simulink library "PCMULib"  (R2022b)
settings: Solver=ode45  StartTime=0.0  StopTime=10.0  RelTol=1e-3  EnableMultiTasking=on
undefined symbols (not defined in the file or in its folder): BreakpointData, BreakpointData1, BreakpointData2, BreakpointData_One_A, BreakpointData_Two_A, caaaa_dbi, caaaa_swi, cTmComprCtrl_n_i16SM4CmpHeatKiMax, cTmComprCtrl_n_i16SM4CmpHeatKiMin, cTmComprCtrl_n_i16SM4CmpHeatKpMax, cTmComprCtrl_n_i16SM4CmpHeatKpMin, cTmComprCtrl_Te_s32ErrCmpPIContinueHeatH, cTmComprCtrl_Te_s32ErrCmpPIContinueHeatL, cTmIn_n_ElacCmprReq_db, cTmIn_n_ElacCmprReq_sw, db, dbi, E2E_P01DataIDMode, E2E_P01ReceiverStatusType, EnumClass, iBit, initalValue, No_Runnable_Period, ObB_EidBsgStDerat_C, p_OVERRIDE_MASTER_SWITCH, SlDemoSign, sw, swi, SwitchOff_P, SwitchOn_P, Table, TableData_M, VCCTi33, VSysD_FidVehDerat1_C
libraries: simulink x22, CCMLib x11, simulink_need_slupdate x9, UXFD_Lib x7, canmsglib x2, PTCC_Lib x1, hdlsllib x1
(part 7 of 7)

== system PCMULib/Standard/Relation&Logic/RS_FF ==
  S : Inport
  R : Inport  Port=2
  AND : Logic  Operator=NOT  Inputs=1  AllPortsSameDT=off  OutDataTypeStr=boolean
  AND1 : Logic  AllPortsSameDT=off  OutDataTypeStr=boolean
  AND2 : Logic  Operator=OR  AllPortsSameDT=off  OutDataTypeStr=boolean
  Unit Delay : UnitDelay  SampleTime=-1  HasFrameUpgradeWarning=on
  Q : Outport
  wires:
  AND/1 -> AND1/1
  R/1 -> AND/1
  S/1 -> AND2/1
  AND2/1 -> AND1/2
  Unit Delay/1 -> AND2/2
  AND1/1 -> Q/1, Unit Delay/1

== system PCMULib/Standard/Relation&Logic/Relay ==
  In2 : Inport
  on : Inport  Port=2
  off : Inport  Port=3
  AND : Logic  Operator=NOT  Inputs=1  AllPortsSameDT=off  OutDataTypeStr=boolean
  AND1 : Logic  Operator=NOT  Inputs=1  AllPortsSameDT=off  OutDataTypeStr=boolean
  AND2 : Logic  AllPortsSameDT=off  OutDataTypeStr=boolean
  AND3 : Logic  Inputs=3  AllPortsSameDT=off  OutDataTypeStr=boolean
  AND4 : Logic  Operator=OR  AllPortsSameDT=off  OutDataTypeStr=boolean
  Relational Operator : RelationalOperator  Operator=<=  OutDataTypeStr=boolean  InputSameDT=off
  Relational Operator1 : RelationalOperator  Operator=<=  OutDataTypeStr=boolean  InputSameDT=off
  Unit Delay : UnitDelay  SampleTime=-1  HasFrameUpgradeWarning=on
  y : Outport
  wires:
  Relational Operator/1 -> AND1/1, AND2/1
  Relational Operator1/1 -> AND/1
  AND3/1 -> AND4/2
  AND4/1 -> Unit Delay/1, y/1
  AND/1 -> AND2/2, AND3/2
  on/1 -> Relational Operator/1
  In2/1 -> Relational Operator1/1, Relational Operator/2
  off/1 -> Relational Operator1/2
  AND2/1 -> AND4/1
  Unit Delay/1 -> AND3/3
  AND1/1 -> AND3/1

== system PCMULib/Standard/Relation&Logic/SignalDelay3 ==
  note: S T E A D Y
  note: D E L A Y
  note: H O L D
  note: T R I G
  note: C O U N T E R
  In1 : Inport
  tdOn : Inport  Port=2
  tdOff : Inport  Port=3
  AND : Logic  Operator=OR  AllPortsSameDT=off  OutDataTypeStr=boolean
  AND1 : Logic  AllPortsSameDT=off  OutDataTypeStr=boolean
  Add : Sum  SaturateOnIntegerOverflow=on
  Constant : Constant  Value=0  OutDataTypeStr=Inherit: Inherit via back propagation
  Constant1 : Constant  Value=0  OutDataTypeStr=Inherit: Inherit via back propagation
  Relational Operator : RelationalOperator  Operator===  OutDataTypeStr=boolean  InputSameDT=off
  Relational Operator1 : RelationalOperator  Operator=>  OutDataTypeStr=boolean  InputSameDT=off
  Relational Operator2 : RelationalOperator  OutDataTypeStr=boolean  InputSameDT=off
  Relational Operator3 : RelationalOperator  Operator===  OutDataTypeStr=boolean  InputSameDT=off
  Switch : Switch  Criteria=u2 ~= 0  Threshold=0.5  SaturateOnIntegerOverflow=off  InputSameDT=off
  Switch1 : Switch  Criteria=u2 ~= 0  Threshold=0.5  SaturateOnIntegerOverflow=off  InputSameDT=off
  Unit Delay : UnitDelay  SampleTime=-1  HasFrameUpgradeWarning=on
  Unit Delay1 : UnitDelay  SampleTime=-1  HasFrameUpgradeWarning=on
  Unit Delay2 : UnitDelay  SampleTime=-1  HasFrameUpgradeWarning=on
  ts : DataStoreRead  DataStoreName=ts  IndexOptions=Index vector (dialog)  Indices=1  OutputSizes=1
  y : Outport
  wires:
  Relational Operator2/1 -> AND/2
  Relational Operator1/1 -> AND1/2
  AND1/1 -> AND/1
  AND/1 -> Unit Delay2/1, Relational Operator3/2
  Unit Delay2/1 -> AND1/1
  Constant1/1 -> Relational Operator1/2
  ts/1 -> Add/2
  Relational Operator3/1 -> y/1
  Switch1/1 -> Relational Operator2/2
  tdOff/1 -> Switch1/3
  Constant/1 -> Switch/3
  Switch/1 -> Unit Delay/1, Relational Operator2/1, Relational Operator1/1
  Unit Delay1/1 -> Relational Operator/1
  In1/1 -> Relational Operator3/1, Unit Delay1/1, Switch1/2, Relational Operator/2
  Add/1 -> Switch/1
  Unit Delay/1 -> Add/1
  Relational Operator/1 -> Switch/2
  tdOn/1 -> Switch1/1

== system PCMULib/Standard/Relation&Logic/SignalTurnOffDelay ==
  note: True = 上面，cnt 清零
      | False = 下面 ，cnt 计数
  note: cnt 计数 < td,保持输出True
  u : Inport
  td : Inport  Port=2
  Add : Sum  SaturateOnIntegerOverflow=on
  Constant : Constant  Value=0
  Delay : Delay  DelayLength=1  InitialConditionSource=Input port  InitialCondition=0
      settings: InputPortMap=u0,p4
  Relational Operator : RelationalOperator  Operator=<=  OutDataTypeStr=boolean  InputSameDT=off
  Switch1 : Switch  Criteria=u2 ~= 0  Threshold=0.5  SaturateOnIntegerOverflow=off  InputSameDT=off
  ts : DataStoreRead  DataStoreName=ts  IndexOptions=Index vector (dialog)  Indices=1  OutputSizes=1
  y : Outport
  wires:
  Constant/1 -> Switch1/1
  Add/1 -> Switch1/3
  Relational Operator/1 -> y/1  "output"
  u/1 -> Switch1/2
  ts/1 -> Add/2
  Delay/1 -> Add/1
  Switch1/1 -> Delay/1, Relational Operator/1  "turnOffCnt"
  td/1 -> Delay/2, Relational Operator/2  "delay_td"

== system PCMULib/Standard/Relation&Logic/SignalTurnOnDelay ==
  u : Inport
  td : Inport  Port=2
  Add : Sum  SaturateOnIntegerOverflow=on
  Constant : Constant  Value=0  OutDataTypeStr=Inherit: Inherit via back propagation
  Relational Operator : RelationalOperator  Operator=>  OutDataTypeStr=boolean  InputSameDT=off
  Switch1 : Switch  Criteria=u2 ~= 0  Threshold=0.5  SaturateOnIntegerOverflow=off  InputSameDT=off
  Unit Delay : UnitDelay  SampleTime=-1  HasFrameUpgradeWarning=on
  ts : DataStoreRead  DataStoreName=ts  IndexOptions=Index vector (dialog)  Indices=1  OutputSizes=1
  y : Outport
  wires:
  ts/1 -> Add/2
  Unit Delay/1 -> Add/1
  td/1 -> Relational Operator/2
  Switch1/1 -> Unit Delay/1, Relational Operator/1
  Add/1 -> Switch1/1
  Constant/1 -> Switch1/3
  u/1 -> Switch1/2
  Relational Operator/1 -> y/1

== system PCMULib/Standard/Relation&Logic/SignalTurnOnOffDelay ==
  note: 1
  note: 0.01
  u : Inport
  td : Inport  Port=2
  Add : Sum  SaturateOnIntegerOverflow=on
  Delay : Delay  DelayLength=1  InitialConditionSource=Input port
      settings: InputPortMap=u0,p4
  Delay1 : Delay  DelayLength=1  InitialConditionSource=Input port
      settings: InputPortMap=u0,p4
  Relational Operator : RelationalOperator  Operator===  OutDataTypeStr=boolean  InputSameDT=off
  Relational Operator1 : RelationalOperator  Operator=>  OutDataTypeStr=boolean  InputSameDT=off
  Switch : Switch  Criteria=u2 ~= 0  Threshold=0.5  OutDataTypeStr=Inherit: Inherit via back propagation  SaturateOnIntegerOverflow=off  InputSameDT=off
  Switch1 : Switch  Criteria=u2 ~= 0  Threshold=0.5  SaturateOnIntegerOverflow=off  InputSameDT=off
  Unit Delay1 : UnitDelay  SampleTime=-1  HasFrameUpgradeWarning=on
  ts : DataStoreRead  DataStoreName=ts  IndexOptions=Index vector (dialog)  Indices=1  OutputSizes=1
  y : Outport
  wires:
  Switch1/1 -> Delay1/1, y/1
  Delay1/1 -> Switch1/3
  Relational Operator1/1 -> Switch1/2
  Relational Operator/1 -> Switch/2
  Add/1 -> Switch/1
  Switch/1 -> Unit Delay1/1, Relational Operator1/1
  td/1 -> Relational Operator1/2
  Unit Delay1/1 -> Add/1
  ts/1 -> Switch/3, Add/2
  u/1 -> Delay/1, Delay/2, Delay1/2, Switch1/1, Relational Operator/1
  Delay/1 -> Relational Operator/2

== system PCMULib/Standard/Relation&Logic/xbackground1 ==

== system PCMULib/Standard/Relation&Logic/xbackground2 ==

== system PCMULib/Standard/Relation&Logic/xbackground3 ==

== system PCMULib/Standard/Relation&Logic/xbackground4 ==

== system PCMULib/Standard/Relation&Logic/xbackground5 ==

== system PCMULib/Standard/Relation&Logic/xbackground6 ==

== system PCMULib/Standard/Relation&Logic/xbackground7 ==

== system PCMULib/Standard/Relation&Logic/xbackground8 ==

== system PCMULib/Standard/Relation&Logic/xbackground9 ==

== system PCMULib/Standard/Signals and systems/ESubsystem ==
  Enable_Name : EnablePort

== system PCMULib/Standard/Signals and systems/ETSubsystem ==
  Enable_Name : EnablePort
  Trigger_Name : TriggerPort  VariantControl=Variant

== system PCMULib/Standard/Signals and systems/Function-Call Subsystem ==
  In1 : Inport
  function : TriggerPort  TriggerType=function-call  VariantControl=Variant
  Out1 : Outport
  wires:
  In1/1 -> Out1/1

== system PCMULib/Standard/Signals and systems/Model Header ==

== system PCMULib/Standard/Signals and systems/RenameSignal ==
  Inport : Inport
  y : Outport
  wires:
  Inport/1 -> y/1

== system PCMULib/Standard/Signals and systems/Subsystem ==
  In1 : Inport
  Out1 : Outport
  wires:
  In1/1 -> Out1/1

== system PCMULib/Standard/Signals and systems/TSubsystem ==
  Trigger_Name : TriggerPort  VariantControl=Variant

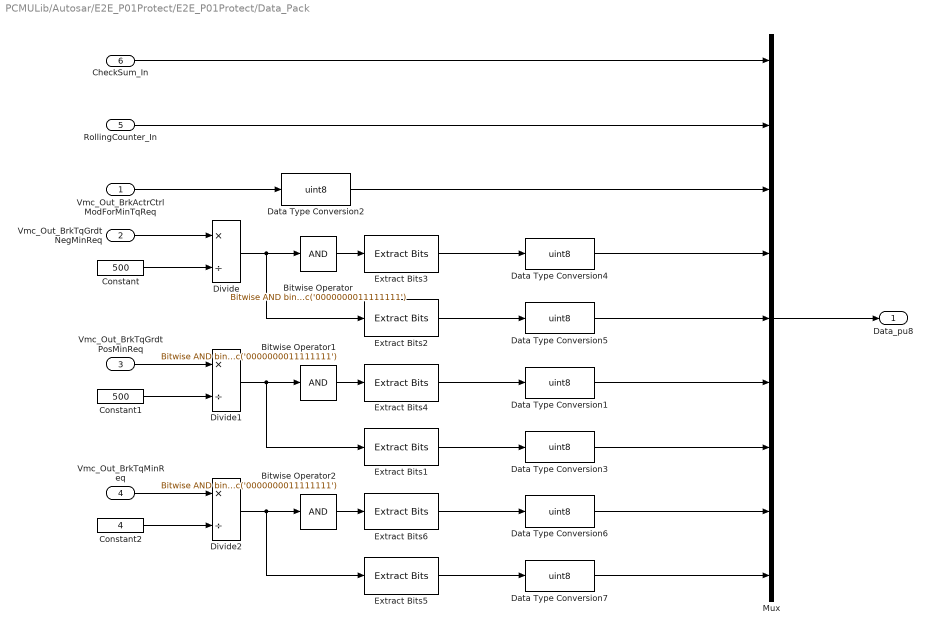
== system PCMULib/Autosar/E2E_P01Protect/E2E_P01Protect/Data_Pack ==
  Vmc_Out_BrkActrCtrlModForMinTqReq : Inport
  Vmc_Out_BrkTqGrdtNegMinReq : Inport  Port=2
  Vmc_Out_BrkTqGrdtPosMinReq : Inport  Port=3
  Vmc_Out_BrkTqMinReq : Inport  Port=4
  RollingCounter_In : Inport  Port=5
  CheckSum_In : Inport  Port=6
  Bitwise Operator : simulink/Logic and Bit Operations/Bitwise Operator  logicop=AND  UseBitMask=on  BitMask=bin2dec('0000000011111111')  BitMaskRealWorld=Stored Integer
  Bitwise Operator1 : simulink/Logic and Bit Operations/Bitwise Operator  logicop=AND  UseBitMask=on  BitMask=bin2dec('0000000011111111')  BitMaskRealWorld=Stored Integer
  Bitwise Operator2 : simulink/Logic and Bit Operations/Bitwise Operator  logicop=AND  UseBitMask=on  BitMask=bin2dec('0000000011111111')  BitMaskRealWorld=Stored Integer
  Constant : Constant  Value=500  OutDataTypeStr=uint16
      settings: CopyFcn=set_param(gcbh,'ShowName','off');
  Constant1 : Constant  Value=500  OutDataTypeStr=uint16
      settings: CopyFcn=set_param(gcbh,'ShowName','off');
  Constant2 : Constant  Value=4  OutDataTypeStr=uint8
      settings: CopyFcn=set_param(gcbh,'ShowName','off');
  Data Type Conversion{1..7} (7 alike) : DataTypeConversion  OutDataTypeStr=uint8  SaturateOnIntegerOverflow=off  RndMeth=Floor
  Divide : Product  Inputs=*/  OutDataTypeStr=uint16
  Divide1 : Product  Inputs=*/  OutDataTypeStr=uint16
  Divide2 : Product  Inputs=*/  OutDataTypeStr=uint16
  Extract Bits1 : simulink/Logic and Bit Operations/Extract Bits  bitsToExtract=Upper half  numBits=8  bitIdxRange=[0 7]  outScalingMode=Treat bit field as an integer
  Extract Bits2 : simulink/Logic and Bit Operations/Extract Bits  bitsToExtract=Upper half  numBits=8  bitIdxRange=[0 7]  outScalingMode=Treat bit field as an integer
  Extract Bits3 : simulink/Logic and Bit Operations/Extract Bits  bitsToExtract=Lower half  numBits=8  bitIdxRange=[0 7]  outScalingMode=Treat bit field as an integer
  Extract Bits4 : simulink/Logic and Bit Operations/Extract Bits  bitsToExtract=Lower half  numBits=8  bitIdxRange=[0 7]  outScalingMode=Treat bit field as an integer
  Extract Bits5 : simulink/Logic and Bit Operations/Extract Bits  bitsToExtract=Upper half  numBits=8  bitIdxRange=[0 7]  outScalingMode=Treat bit field as an integer
  Extract Bits6 : simulink/Logic and Bit Operations/Extract Bits  bitsToExtract=Lower half  numBits=8  bitIdxRange=[0 7]  outScalingMode=Treat bit field as an integer
  Mux : Mux  Inputs=9
  Data_pu8 : Outport
  wires:
  Mux/1 -> Data_pu8/1
  Vmc_Out_BrkActrCtrlModForMinTqReq/1 -> Data Type Conversion2/1
  Extract Bits3/1 -> Data Type Conversion4/1
  Constant/1 -> Divide/2
  Bitwise Operator/1 -> Extract Bits3/1
  Extract Bits2/1 -> Data Type Conversion5/1
  Divide/1 -> Extract Bits2/1, Bitwise Operator/1
  Vmc_Out_BrkTqGrdtNegMinReq/1 -> Divide/1
  Extract Bits4/1 -> Data Type Conversion1/1
  Constant1/1 -> Divide1/2
  Bitwise Operator1/1 -> Extract Bits4/1
  Extract Bits1/1 -> Data Type Conversion3/1
  Divide1/1 -> Extract Bits1/1, Bitwise Operator1/1
  Vmc_Out_BrkTqGrdtPosMinReq/1 -> Divide1/1
  Extract Bits6/1 -> Data Type Conversion6/1
  Constant2/1 -> Divide2/2
  Bitwise Operator2/1 -> Extract Bits6/1
  Extract Bits5/1 -> Data Type Conversion7/1
  Divide2/1 -> Extract Bits5/1, Bitwise Operator2/1
  Vmc_Out_BrkTqMinReq/1 -> Divide2/1
  RollingCounter_In/1 -> Mux/2
  CheckSum_In/1 -> Mux/1
  Data Type Conversion2/1 -> Mux/3
  Data Type Conversion4/1 -> Mux/4
  Data Type Conversion5/1 -> Mux/5
  Data Type Conversion1/1 -> Mux/6
  Data Type Conversion3/1 -> Mux/7
  Data Type Conversion6/1 -> Mux/8
  Data Type Conversion7/1 -> Mux/9

== system PCMULib/Autosar/E2E_P01Protect/E2E_P01Protect/E2E_Config ==
  DataLength : Inport
  DataID : Inport  Port=2
  BusCreator : BusCreator  Inputs=6  OutDataTypeStr=Bus: E2E_P01ConfigType  NonVirtualBus=on
      settings: CopyFcn=set_param(gcbh,'ShowName','off');  InheritFromInputs=off
  CRCOffset : Constant  Value=0  OutDataTypeStr=uint16
  CounterOffset : Constant  Value=8  OutDataTypeStr=uint16
  DataIDMode : simulink/Sources/Enumerated Constant  OutDataTypeStr=Enum: E2E_P01DataIDMode  Value=E2E_P01DataIDMode.E2E_P01_DATAID_BOTH  SampleTime=inf
  MaxDeltaCounterInit : Constant  Value=14  OutDataTypeStr=uint8
  E2E_P01_Config : Outport
  wires:
  DataID/1 -> BusCreator/2
  CounterOffset/1 -> BusCreator/6
  MaxDeltaCounterInit/1 -> BusCreator/4
  BusCreator/1 -> E2E_P01_Config/1
  DataIDMode/1 -> BusCreator/3
  DataLength/1 -> BusCreator/1
  CRCOffset/1 -> BusCreator/5

== system PCMULib/Autosar/E2E_P01Protect/E2E_P01Protect/E2E_P01Protect_S ==
  ConfigType : Inport
  SenderStateType : Inport  Port=2
  Data_pu8 : Inport  Port=3
  S-Function : S-Function  FunctionName=E2E_P01Protect_S  SFunctionDeploymentMode=off  EnableBusSupport=off
  Std_ReturnType : Outport
  wires:
  S-Function/1 -> Std_ReturnType/1
  Data_pu8/1 -> S-Function/3
  ConfigType/1 -> S-Function/1
  SenderStateType/1 -> S-Function/2

== system PCMULib/Autosar/E2E_P01_Check/E2E_Check/E2E_Check ==
  Status : Inport
  DataLength : Inport  Port=2
  DataID : Inport  Port=3
  AccrPedlNotCmpl_IsUpdated : Inport  Port=4
  CheckSum : Inport  Port=5
  RollingCounter : Inport  Port=6
  AccrPedlNotCmpl_Psd : Inport  Port=7
  AccrPedlNotCmpl_PsdSts : Inport  Port=8
  Data_ID_218 : Subsystem
  E2E_Config_ID_218 : Subsystem
  E2E_P01Check_S : Subsystem
      mask Display:
      | disp('E2E_P01Check');
      | port_label('input',1,'ConfigType');
      | port_label('input',2,'ReceiverStateType');
      | port_label('input',3,'Data_pu8');
      | port_label('output',1,'Std_ReturnType');
  E2E_P01ReceiverID_218 : Subsystem
  E2E_P01Check_ReturnType : Outport
  E2E_P01ReceiverStatus : Outport  Port=2
  wires:
  RollingCounter/1 -> Data_ID_218/2(RollingCounter)
  CheckSum/1 -> Data_ID_218/1(CheckSum)
  Data_ID_218/1(Data_pu8) -> E2E_P01Check_S/3(Data_pu8)
  E2E_P01Check_S/1(Std_ReturnType) -> E2E_P01Check_ReturnType/1
  E2E_Config_ID_218/1(E2E_Config_ID_218) -> E2E_P01Check_S/1(ConfigType)
  AccrPedlNotCmpl_IsUpdated/1 -> E2E_P01ReceiverID_218/1(AccrPedlNotCmpl_IsUpdated)
  DataLength/1 -> E2E_Config_ID_218/1(DataLength)
  E2E_P01ReceiverID_218/1(E2E_P01ReceiverState) -> E2E_P01ReceiverStatus/1, E2E_P01Check_S/2(ReceiverStateType)
  DataID/1 -> E2E_Config_ID_218/2(DataID)
  Status/1 -> E2E_P01ReceiverID_218/2(Status)
  AccrPedlNotCmpl_Psd/1 -> Data_ID_218/3(AccrPedlNotCmpl_Psd)
  AccrPedlNotCmpl_PsdSts/1 -> Data_ID_218/4(AccrPedlNotCmpl_PsdSts)

== system PCMULib/Calculation/PI/SaturationAndDeadband/absolute ==
  Input : Inport
  Compare To Constant2 : simulink/Logic and Bit Operations/Compare To Constant  relop=>=  const=0  OutDataTypeStr=boolean
  Constant10 : Constant  Value=0  OutDataTypeStr=Inherit: Inherit via back propagation
  Subtract : Sum  Inputs=-+  OutDataTypeStr=Inherit: Inherit via back propagation
  Switch10 : Switch  Criteria=u2 > Threshold  SaturateOnIntegerOverflow=off  InputSameDT=off
  Output : Outport  VectorParamsAs1DForOutWhenUnconnected=off
  wires:
  Constant10/1 -> Subtract/2
  Input/1 -> Subtract/1, Compare To Constant2/1, Switch10/1
  Subtract/1 -> Switch10/3
  Switch10/1 -> Output/1
  Compare To Constant2/1 -> Switch10/2

== system PCMULib/Custom/CAN/CanHex2Signed/condtion ==
  note: 判断条件:2^(n-1)-1
  note: 模：2^n
  bitL : Inport
  Add : Sum  Inputs=+-
      settings: CopyFcn=set_param(gcbh,'ShowName','off');
  Add1 : Sum  Inputs=+-
      settings: CopyFcn=set_param(gcbh,'ShowName','off');
  Constant : Constant  Value=2  OutDataTypeStr=single
      settings: CopyFcn=set_param(gcbh,'ShowName','off');
  Constant1 : Constant  OutDataTypeStr=single
      settings: CopyFcn=set_param(gcbh,'ShowName','off');
  Constant3 : Constant  OutDataTypeStr=uint8
      settings: CopyFcn=set_param(gcbh,'ShowName','off');
  Constant4 : Constant  Value=2  OutDataTypeStr=single
      settings: CopyFcn=set_param(gcbh,'ShowName','off');
  Gain : Gain  OutDataTypeStr=uint32
      settings: CopyFcn=set_param(gcbh,'ShowName','off');
  Math Function : Math  Operator=pow  SignedPower=on  OutputSignalType=real
  Math Function1 : Math  Operator=pow  SignedPower=on  OutputSignalType=real
  cond : Outport
  2^n : Outport  Port=2
  wires:
  Add/1 -> cond/1
  Gain/1 -> Add/1
  Constant4/1 -> Math Function1/1
  Add1/1 -> Math Function1/2
  Constant1/1 -> Add1/2
  Constant/1 -> Math Function/1
  Math Function/1 -> 2^n/1
  Math Function1/1 -> Gain/1
  Constant3/1 -> Add/2
  bitL/1 -> Math Function/2, Add1/1

== system PCMULib/Custom/CAN/CanHex2Signed/signal_conditioning ==
  note: 判断输入的BitLength是否（0<u1<=32bit）;
      | 并向下取整。
  In1 : Inport
  Constant1 : Constant  Value=0  OutDataTypeStr=single
      settings: CopyFcn=set_param(gcbh,'ShowName','off');
  Constant2 : Constant  Value=32  OutDataTypeStr=single
      settings: CopyFcn=set_param(gcbh,'ShowName','off');
  Constant4 : Constant  Value=32  OutDataTypeStr=single
      settings: CopyFcn=set_param(gcbh,'ShowName','off');
  Constant7 : Constant  Value=0  OutDataTypeStr=single
      settings: CopyFcn=set_param(gcbh,'ShowName','off');
  Floor : Subsystem  mask(GL_Floor){}
      mask help: Floor block rounds the input variable to the nearest integer towards minus infinity.
      mask init:
      | set_param(gcb,'LinkStatus','none');
      settings: CopyFcn=set_param(gcbh,'ShowName','off');
      mask Display: text(0.1,0.5, 'Floor')
  Relational Operator1 : RelationalOperator  Operator=<  OutDataTypeStr=boolean  InputSameDT=off
  Relational Operator2 : RelationalOperator  Operator=>  OutDataTypeStr=boolean  InputSameDT=off
  Switch : Switch  Criteria=u2 > Threshold  SaturateOnIntegerOverflow=off  InputSameDT=off
  Switch1 : Switch  Criteria=u2 > Threshold  SaturateOnIntegerOverflow=off  InputSameDT=off
  BitLength_BeUsed : Outport
  wires:
  Floor/1(Out1) -> Switch1/1
  Relational Operator2/1 -> Switch/2
  Constant1/1 -> Relational Operator2/2
  Relational Operator1/1 -> Switch1/2
  Switch/1 -> Floor/1(In1), Relational Operator1/1
  Constant4/1 -> Relational Operator1/2
  Constant2/1 -> Switch1/3
  Switch1/1 -> BitLength_BeUsed/1
  Constant7/1 -> Switch/3
  In1/1 -> Relational Operator2/1, Switch/1

== system PCMULib/Custom/CAN/CanHex2Signed/value<0 ==
  hex : Inport
  2^n : Inport  Port=2  OutDataTypeStr=single
  Action Port : ActionPort
  Add : Sum  Inputs=+-
      settings: CopyFcn=set_param(gcbh,'ShowName','off');
  Gain1 : Gain  OutDataTypeStr=single
      settings: CopyFcn=set_param(gcbh,'ShowName','off');
  Gain8 : Gain  OutDataTypeStr=single
      settings: CopyFcn=set_param(gcbh,'ShowName','off');
  Out1 : Outport
  wires:
  Gain1/1 -> Add/2
  2^n/1 -> Gain1/1
  Gain8/1 -> Out1/1
  Add/1 -> Gain8/1
  hex/1 -> Add/1

== system PCMULib/Custom/CAN/CanHex2Signed/value>0 ==
  hex : Inport
  Action Port : ActionPort
  Gain9 : Gain  OutDataTypeStr=single
      settings: CopyFcn=set_param(gcbh,'ShowName','off');
  Out1 : Outport
  wires:
  Gain9/1 -> Out1/1
  hex/1 -> Gain9/1

== system PCMULib/Custom/Diagnose/Dem_SetEventStatus/Dem_SetEventStatus_Enable ==
  EventID : Inport
  EveSt : Inport  Port=2
  Enable : EnablePort
  Dem_SetEventStatus_Asw : S-Function  FunctionName=Dem_SetEventStatus_Asw_SF  SFunctionDeploymentMode=off  EnableBusSupport=off  mask(Legacy Function){SFunctionSpec=void Dem_SetEventStatus_Asw(uint16 u1, uint8 u2), ShowSpec=on}
      mask prompts: ShowSpec "Display function specification"
      mask help:
      | This block allows you to call the legacy functions specified by the following Legacy Code Tool definition:
      | def.SFunctionName = 'Dem_SetEventStatus_Asw_SF';
      | def.OutputFcnSpec = 'void Dem_SetEventStatus_Asw(uint16 u1, uint8 u2)';
      | def.HeaderFiles = {'Dem.h'};
      | def.SourceFiles = {'Dem.c'};
      mask Help: <p>This block was generated automatically by the Legacy Code Tool. For detailed help on this tool, call<a href="matlab:legacy_code('help')"> legacy_code('help')</a>.</p>
      mask Callback ShowSpec:
      | if strcmp(get_param(gcbh, 'ShowSpec'), 'on')
      |   set_param(gcbh, 'MaskDisplay', sprintf('fprintf(''%s'');', get_param(gcbh, 'SFunctionSpec')));
      | else
      |   set_param(gcbh, 'MaskDisplay', sprintf('fprintf(''%s'');', get_param(gcbh, 'FunctionName')));
      | end
      mask Display: fprintf('void Dem_SetEventStatus_Asw(uint16 u1, uint8 u2)');
  wires:
  EveSt/1 -> Dem_SetEventStatus_Asw/2
  EventID/1 -> Dem_SetEventStatus_Asw/1

== system PCMULib/Standard/Discrete dynamics/BumplessRateTransfer/LogicalSwitch1 ==
  In1 : Inport
  In2 : Inport  Port=2
  In3 : Inport  Port=3
  Switch : Switch  Criteria=u2 > Threshold  Threshold=0.5  SaturateOnIntegerOverflow=off  InputSameDT=off
  Out1 : Outport
  wires:
  In1/1 -> Switch/1
  In3/1 -> Switch/2
  In2/1 -> Switch/3
  Switch/1 -> Out1/1

== system PCMULib/Standard/Discrete dynamics/BumplessRateTransfer/RateLimit ==
  In1 : Inport
  dr : Inport  Port=2
  df : Inport  Port=3
  Abs : Abs  SaturateOnIntegerOverflow=off
  Add : Sum  Inputs=+-
  Add1 : Sum
  MinMax : MinMax  Function=max  Inputs=2
  MinMax1 : MinMax  Inputs=2
  Product : Product
  Product1 : Product
  Subsystem1 : Subsystem
      mask help:
      | this block use for the situation when the first run use the Initail Value , after the first run , use the CalValue.
      | output is the Initial Value when first run ; otherwise is the calValue.
      mask Display: dpoly([0 0 1], [0 1 0], 'z')
  ts : DataStoreRead  DataStoreName=ts  IndexOptions=Index vector (dialog)  Indices=1  OutputSizes=1
  y : Outport
  wires:
  In1/1 -> Subsystem1/1(InitialValue), MinMax/1
  Add1/1 -> MinMax1/2
  dr/1 -> Product1/2
  MinMax1/1 -> Subsystem1/2(CalValue), y/1
  Product1/1 -> Add1/2
  MinMax/1 -> MinMax1/1
  Add/1 -> MinMax/2
  Product/1 -> Abs/1
  df/1 -> Product/2
  ts/1 -> Product1/1, Product/1
  Abs/1 -> Add/2
  Subsystem1/1(Output) -> Add1/1, Add/1

== system PCMULib/Standard/Discrete dynamics/BumplessTransfer/LPF1_pole1 ==
  u : Inport
  tc : Inport  Port=2
  Add : Sum  Inputs=-+
  Add1 : Sum
  Constant : Constant  Value=1e-6  OutDataTypeStr=single
  Divide : Product  Inputs=*/
  MinMax : MinMax  Function=max  Inputs=3
  Product : Product
  Subsystem1 : Subsystem
      mask help:
      | this block use for the situation when the first run use the Initail Value , after the first run , use the CalValue.
      | output is the Initial Value when first run ; otherwise is the calValue.
      mask Display: dpoly([0 0 1], [0 1 0], 'z')
  ts : DataStoreRead  DataStoreName=ts  IndexOptions=Index vector (dialog)  Indices=1  OutputSizes=1
  y : Outport
  wires:
  Add1/1 -> Subsystem1/2(CalValue), y/1
  u/1 -> Subsystem1/1(InitialValue), Add/2
  Add/1 -> Product/1
  MinMax/1 -> Divide/2
  tc/1 -> MinMax/2
  ts/1 -> Divide/1, MinMax/1
  Divide/1 -> Product/2
  Subsystem1/1(Output) -> Add/1, Add1/1
  Product/1 -> Add1/2
  Constant/1 -> MinMax/3

== system PCMULib/Standard/Discrete dynamics/BumplessTransfer/LogicalSwitch1 ==
  In1 : Inport
  In2 : Inport  Port=2
  In3 : Inport  Port=3
  Switch : Switch  Criteria=u2 > Threshold  Threshold=0.5  SaturateOnIntegerOverflow=off  InputSameDT=off
  Out1 : Outport
  wires:
  In1/1 -> Switch/1
  In3/1 -> Switch/2
  In2/1 -> Switch/3
  Switch/1 -> Out1/1

== system PCMULib/Standard/Discrete dynamics/DLPF1_pole_v2/LogicalSwitch1 ==
  In1 : Inport
  In2 : Inport  Port=2
  In3 : Inport  Port=3
  Switch : Switch  Criteria=u2 > Threshold  Threshold=0.5  SaturateOnIntegerOverflow=off  InputSameDT=off
  Out1 : Outport
  wires:
  In1/1 -> Switch/1
  In3/1 -> Switch/2
  In2/1 -> Switch/3
  Switch/1 -> Out1/1

== system PCMULib/Standard/Discrete dynamics/HysteresisFilter/Saturation1 ==
  u : Inport
  U : Inport  Port=2
  L : Inport  Port=3
  MinMax : MinMax  Inputs=2
  MinMax1 : MinMax  Function=max  Inputs=2
  y : Outport
  wires:
  L/1 -> MinMax1/2
  MinMax1/1 -> y/1
  u/1 -> MinMax/2
  U/1 -> MinMax/1
  MinMax/1 -> MinMax1/1

== system PCMULib/Standard/Discrete dynamics/LPF1_discreteReset/LogicalSwitch1 ==
  In1 : Inport
  In3 : Inport  Port=2
  In2 : Inport  Port=3
  Switch : Switch  Criteria=u2 ~= 0  Threshold=0.5  mask(TL_Switch){data={'logdata',{'maxnumvals',4096,'plotchannels',[]},'output',{'type','Float32'},'date',735300.29228125}}
      settings: CopyFcn=if exist('tl_reset_reviewflag','file')==2,tl_reset_reviewflag(gcbh);end  DeleteFcn=if exist('delete_tlblock','file')==2,delete_tlblock(gcbh);end  NameChangeFcn=if exist('rename_tlblock','file')==2,rename_tlblock(gcbh);end  OpenFcn=if exist('tl_open_blockdlg','file')==2,tl_open_blockdlg(gcbh);else,open_system(gcbh,'parameter');end
      mask Help: eval(['if exist(''tl_online_help'',''file'') == 2, tl_online_help(''Topic'',''TL_Switch''),else, web([''jar:file:///'',matlabroot,''/help/toolbox/simulink/help.jar!/slref/' lower(get_param(gcbh,'Blocktype')) '.html''], ''-helpbrowser''),end'])
      mask Display: plot([-0.05, 1.05, NaN, -0.05, 1.05],[.01, .01, NaN, .99, .99])
  Out1 : Outport
  wires:
  In1/1 -> Switch/1
  In2/1 -> Switch/2
  In3/1 -> Switch/3
  Switch/1 -> Out1/1

== system PCMULib/Standard/Math/Floor/mod1 ==
  In1 : Inport
  In2 : Inport  Port=2
  Mod : Math  Operator=mod  SignedPower=on
  Out1 : Outport
  wires:
  In1/1 -> Mod/1
  Mod/1 -> Out1/1
  In2/1 -> Mod/2

== system PCMULib/Standard/Math/Interpolation/Safe_Divide ==
  In3 : Inport
  In2 : Inport  Port=2
  In1 : Inport  Port=3
  Constant : Constant  Value=0  OutDataTypeStr=Inherit: Inherit via back propagation
  Gain : Gain  Gain=-1
  LogicalSwitch : Subsystem  mask(PAG_Switch_LV1.6_BV2){}
      mask help:
      | Pass through input 1 when input 3 is true;
      | otherwise, pass through input 2
      mask Display:
      | plot([-0.1 0.2 0.2], [0.85 0.85 0.75])
      | plot([-0.1 0.2 0.2], [0.5 0.5 0.6])
      | plot([0.8 1.1], [0.5 0.5])
      | plot([0.15 0.8], [0.6 0.5])
      | plot([-0.1 0.5 0.5], [0.15 0.15 0.6])
  Max : MinMax  Function=max  Inputs=2
  MinMax : MinMax  Inputs=2
  Product1 : Product  Inputs=*/
  Relational Operator : RelationalOperator  Operator=<  OutDataTypeStr=boolean  InputSameDT=off
  Out1 : Outport
  wires:
  Constant/1 -> Relational Operator/2
  Relational Operator/1 -> LogicalSwitch/3(In3)
  MinMax/1 -> LogicalSwitch/1(In1)
  In1/1 -> Gain/1, Max/1
  In2/1 -> Relational Operator/1, Max/2, MinMax/1
  Max/1 -> LogicalSwitch/2(In2)
  In3/1 -> Product1/1
  Product1/1 -> Out1/1
  Gain/1 -> MinMax/2
  LogicalSwitch/1(Out1) -> Product1/2

== system PCMULib/Standard/Math/LimitInterpolation/Safe_Divide ==
  In3 : Inport
  In2 : Inport  Port=2
  In1 : Inport  Port=3
  Constant : Constant  Value=0  OutDataTypeStr=Inherit: Inherit via back propagation
  Gain : Gain  Gain=-1
  LogicalSwitch : Subsystem  mask(PAG_Switch_LV1.6_BV2){}
      mask help:
      | Pass through input 1 when input 3 is true;
      | otherwise, pass through input 2
      mask Display:
      | plot([-0.1 0.2 0.2], [0.85 0.85 0.75])
      | plot([-0.1 0.2 0.2], [0.5 0.5 0.6])
      | plot([0.8 1.1], [0.5 0.5])
      | plot([0.15 0.8], [0.6 0.5])
      | plot([-0.1 0.5 0.5], [0.15 0.15 0.6])
  Max : MinMax  Function=max  Inputs=2
  MinMax : MinMax  Inputs=2
  Product1 : Product  Inputs=*/
  Relational Operator : RelationalOperator  Operator=<  OutDataTypeStr=boolean  InputSameDT=off
  Out1 : Outport
  wires:
  Constant/1 -> Relational Operator/2
  Relational Operator/1 -> LogicalSwitch/3(In3)
  MinMax/1 -> LogicalSwitch/1(In1)
  In1/1 -> Gain/1, Max/1
  In2/1 -> Relational Operator/1, Max/2, MinMax/1
  Max/1 -> LogicalSwitch/2(In2)
  In3/1 -> Product1/1
  Product1/1 -> Out1/1
  Gain/1 -> MinMax/2
  LogicalSwitch/1(Out1) -> Product1/2

== system PCMULib/Standard/Math/LimitInterpolation/Saturation ==
  u : Inport
  U : Inport  Port=2
  L : Inport  Port=3
  MinMax : MinMax  Inputs=2
  MinMax1 : MinMax  Function=max  Inputs=2
  y : Outport
  wires:
  MinMax/1 -> MinMax1/1
  U/1 -> MinMax/1
  u/1 -> MinMax/2
  MinMax1/1 -> y/1
  L/1 -> MinMax1/2

== system PCMULib/Standard/Math/Round/mod ==
  In1 : Inport
  In2 : Inport  Port=2
  mod : Subsystem  mask(GL_Mod_1.0){}
      mask help: Signed remainder after division.
      mask Display: disp('mod')
  Out1 : Outport
  wires:
  In1/1 -> mod/1(In1)
  mod/1(Out1) -> Out1/1
  In2/1 -> mod/2(In2)

== system PCMULib/Standard/Math/Safe_Divide/LogicalSwitch ==
  In1 : Inport
  In2 : Inport  Port=2
  In3 : Inport  Port=3
  Switch : Switch  Criteria=u2 ~= 0  Threshold=1  OutDataTypeStr=Inherit: Inherit via back propagation  RndMeth=Round
      settings: AttributesFormatString=%<Criteria>  CopyFcn=set_param(gcbh,'ShowName','off');
  Out1 : Outport
  wires:
  In1/1 -> Switch/1
  In3/1 -> Switch/2
  In2/1 -> Switch/3
  Switch/1 -> Out1/1

== system PCMULib/Autosar/E2E_P01_Check/E2E_Check/E2E_Check/Data_ID_218 ==
  CheckSum : Inport
  RollingCounter : Inport  Port=2
  AccrPedlNotCmpl_Psd : Inport  Port=3
  AccrPedlNotCmpl_PsdSts : Inport  Port=4
  Data Type Conversion{1..2,4..5} (4 alike) : DataTypeConversion  OutDataTypeStr=uint8  SaturateOnIntegerOverflow=off  RndMeth=Floor
  Data Type Conversion6 : DataTypeConversion  SaturateOnIntegerOverflow=off  RndMeth=Floor
  Mux2 : Mux
  Data_pu8 : Outport
  wires:
  Data Type Conversion4/1 -> Mux2/3
  Data Type Conversion5/1 -> Mux2/4
  Mux2/1 -> Data Type Conversion6/1
  Data Type Conversion6/1 -> Data_pu8/1
  RollingCounter/1 -> Data Type Conversion1/1
  CheckSum/1 -> Data Type Conversion2/1
  AccrPedlNotCmpl_PsdSts/1 -> Data Type Conversion5/1
  AccrPedlNotCmpl_Psd/1 -> Data Type Conversion4/1
  Data Type Conversion1/1 -> Mux2/2
  Data Type Conversion2/1 -> Mux2/1

== system PCMULib/Autosar/E2E_P01_Check/E2E_Check/E2E_Check/E2E_Config_ID_218 ==
  DataLength : Inport
  DataID : Inport  Port=2
  BusCreator2 : BusCreator  Inputs=6  OutDataTypeStr=Bus: E2E_P01ConfigType  NonVirtualBus=on
      settings: CopyFcn=set_param(gcbh,'ShowName','off');  InheritFromInputs=off
  CRCOffset : Constant  Value=0  OutDataTypeStr=uint16
  CounterOffset : Constant  Value=8  OutDataTypeStr=uint16
  DataIDMode : simulink/Sources/Enumerated Constant  OutDataTypeStr=Enum: E2E_P01DataIDMode  Value=E2E_P01DataIDMode.E2E_P01_DATAID_BOTH  SampleTime=inf
  MaxDeltaCounterInit : Constant  Value=14  OutDataTypeStr=uint8
  E2E_Config_ID_218 : Outport
  wires:
  CounterOffset/1 -> BusCreator2/6
  DataLength/1 -> BusCreator2/1
  MaxDeltaCounterInit/1 -> BusCreator2/4
  BusCreator2/1 -> E2E_Config_ID_218/1
  CRCOffset/1 -> BusCreator2/5
  DataID/1 -> BusCreator2/2
  DataIDMode/1 -> BusCreator2/3

== system PCMULib/Autosar/E2E_P01_Check/E2E_Check/E2E_Check/E2E_P01Check_S ==
  ConfigType : Inport
  ReceiverStateType : Inport  Port=2
  Data_pu8 : Inport  Port=3
  S-Function : S-Function  FunctionName=E2E_P01Check_S  SFunctionDeploymentMode=off  EnableBusSupport=off
  Std_ReturnType : Outport
  wires:
  S-Function/1 -> Std_ReturnType/1
  Data_pu8/1 -> S-Function/3
  ConfigType/1 -> S-Function/1
  ReceiverStateType/1 -> S-Function/2

== system PCMULib/Autosar/E2E_P01_Check/E2E_Check/E2E_Check/E2E_P01ReceiverID_218 ==
  AccrPedlNotCmpl_IsUpdated : Inport  OutDataTypeStr=boolean
  Status : Inport  Port=2
  BusCreator3 : BusCreator  Inputs=6  OutDataTypeStr=Bus: E2E_P01ReceiverStateType  NonVirtualBus=on
      settings: CopyFcn=set_param(gcbh,'ShowName','off');  InheritFromInputs=off
  LastValidCounter : Constant  Value=0  OutDataTypeStr=uint8
  LostData : Constant  Value=0  OutDataTypeStr=uint8
  MaxDeltaCounter : Constant  Value=0  OutDataTypeStr=uint8
  WaitForFirstData : Constant  OutDataTypeStr=boolean
  E2E_P01ReceiverState : Outport
  wires:
  LastValidCounter/1 -> BusCreator3/1
  WaitForFirstData/1 -> BusCreator3/3
  MaxDeltaCounter/1 -> BusCreator3/2
  LostData/1 -> BusCreator3/5
  BusCreator3/1 -> E2E_P01ReceiverState/1
  AccrPedlNotCmpl_IsUpdated/1 -> BusCreator3/4
  Status/1 -> BusCreator3/6

== system PCMULib/Custom/CAN/CanHex2Signed/signal_conditioning/Floor ==
  In1 : Inport
  Add : Sum  Inputs=+-
  Constant : Constant  OutDataTypeStr=single
  mod1 : Subsystem  mask(GL_Mod_1.0){}
      mask help: Signed remainder after division.
      mask Display: disp('mod')
  Out1 : Outport
  wires:
  Constant/1 -> mod1/2(In2)
  Add/1 -> Out1/1
  In1/1 -> mod1/1(In1), Add/1
  mod1/1(Out1) -> Add/2

== system PCMULib/Standard/Discrete dynamics/BumplessRateTransfer/RateLimit/Subsystem1 ==
  InitialValue : Inport
  CalValue : Inport  Port=2
  Constant12 : Constant  Value=0
      settings: CopyFcn=set_param(gcbh,'ShowName','off');
  ESubsystem : Subsystem  TreatAsAtomicUnit=on
      mask init:
      | set_param(gcb, 'LinkStatus', 'none');
      mask Display: disp(' ');
  Relational Operator10 : RelationalOperator  Operator===  OutDataTypeStr=boolean  InputSameDT=off
      settings: CopyFcn=set_param(gcbh,'ShowName','off');
  Switch1 : Switch  Criteria=u2 ~= 0  Threshold=1  OutDataTypeStr=Inherit: Inherit via back propagation  RndMeth=Round
      settings: AttributesFormatString=%<Criteria>  CopyFcn=set_param(gcbh,'ShowName','off');
  Unit Delay : UnitDelay  SampleTime=-1  HasFrameUpgradeWarning=on
      settings: CopyFcn=set_param(gcbh,'ShowName','off');
  Unit Delay1 : UnitDelay  SampleTime=-1  HasFrameUpgradeWarning=on
      settings: CopyFcn=set_param(gcbh,'ShowName','off');
  Output : Outport
  wires:
  Constant12/1 -> Relational Operator10/2
  ESubsystem/1(Out1) -> Unit Delay/1
  Unit Delay/1 -> Relational Operator10/1
  Relational Operator10/1 -> Switch1/2, ESubsystem/Enable
  InitialValue/1 -> Switch1/1
  CalValue/1 -> Unit Delay1/1
  Switch1/1 -> Output/1
  Unit Delay1/1 -> Switch1/3

== system PCMULib/Standard/Discrete dynamics/BumplessTransfer/LPF1_pole1/Subsystem1 ==
  InitialValue : Inport
  CalValue : Inport  Port=2
  Constant12 : Constant  Value=0
      settings: CopyFcn=set_param(gcbh,'ShowName','off');
  ESubsystem : Subsystem  TreatAsAtomicUnit=on
      mask init:
      | set_param(gcb, 'LinkStatus', 'none');
      mask Display: disp(' ');
  Relational Operator10 : RelationalOperator  Operator===  OutDataTypeStr=boolean  InputSameDT=off
      settings: CopyFcn=set_param(gcbh,'ShowName','off');
  Switch1 : Switch  Criteria=u2 ~= 0  Threshold=1  OutDataTypeStr=Inherit: Inherit via back propagation  RndMeth=Round
      settings: AttributesFormatString=%<Criteria>  CopyFcn=set_param(gcbh,'ShowName','off');
  Unit Delay : UnitDelay  SampleTime=-1  HasFrameUpgradeWarning=on
      settings: CopyFcn=set_param(gcbh,'ShowName','off');
  Unit Delay1 : UnitDelay  SampleTime=-1  HasFrameUpgradeWarning=on
      settings: CopyFcn=set_param(gcbh,'ShowName','off');
  Output : Outport
  wires:
  Constant12/1 -> Relational Operator10/2
  ESubsystem/1(Out1) -> Unit Delay/1
  Unit Delay/1 -> Relational Operator10/1
  Relational Operator10/1 -> Switch1/2, ESubsystem/Enable
  InitialValue/1 -> Switch1/1
  CalValue/1 -> Unit Delay1/1
  Switch1/1 -> Output/1
  Unit Delay1/1 -> Switch1/3

== system PCMULib/Standard/Math/Interpolation/Safe_Divide/LogicalSwitch ==
  In1 : Inport
  In2 : Inport  Port=2
  In3 : Inport  Port=3
  Switch : Switch  Threshold=0.5  mask(TL_Switch){data={'logdata',{'maxnumvals',4096,'plotchannels',[]},'output',{'type','Float32'},'date',735300.29223627318}}
      settings: CopyFcn=if exist('tl_reset_reviewflag','file')==2,tl_reset_reviewflag(gcbh);end  DeleteFcn=if exist('delete_tlblock','file')==2,delete_tlblock(gcbh);end  NameChangeFcn=if exist('rename_tlblock','file')==2,rename_tlblock(gcbh);end  OpenFcn=if exist('tl_open_blockdlg','file')==2,tl_open_blockdlg(gcbh);else,open_system(gcbh,'parameter');end
      mask Help: eval(['if exist(''tl_online_help'',''file'') == 2, tl_online_help(''Topic'',''TL_Switch''),else, web([''jar:file:///'',matlabroot,''/help/toolbox/simulink/help.jar!/slref/' lower(get_param(gcbh,'Blocktype')) '.html''], ''-helpbrowser''),end'])
      mask Display: plot([-0.05, 1.05, NaN, -0.05, 1.05],[.01, .01, NaN, .99, .99])
  Out1 : Outport
  wires:
  Switch/1 -> Out1/1
  In2/1 -> Switch/3
  In3/1 -> Switch/2
  In1/1 -> Switch/1

== system PCMULib/Standard/Math/LimitInterpolation/Safe_Divide/LogicalSwitch ==
  In1 : Inport
  In2 : Inport  Port=2
  In3 : Inport  Port=3
  Switch : Switch  Threshold=0.5  mask(TL_Switch){data={'logdata',{'maxnumvals',4096,'plotchannels',[]},'output',{'type','Float32'},'date',735300.29223627318}}
      settings: CopyFcn=if exist('tl_reset_reviewflag','file')==2,tl_reset_reviewflag(gcbh);end  DeleteFcn=if exist('delete_tlblock','file')==2,delete_tlblock(gcbh);end  NameChangeFcn=if exist('rename_tlblock','file')==2,rename_tlblock(gcbh);end  OpenFcn=if exist('tl_open_blockdlg','file')==2,tl_open_blockdlg(gcbh);else,open_system(gcbh,'parameter');end
      mask Help: eval(['if exist(''tl_online_help'',''file'') == 2, tl_online_help(''Topic'',''TL_Switch''),else, web([''jar:file:///'',matlabroot,''/help/toolbox/simulink/help.jar!/slref/' lower(get_param(gcbh,'Blocktype')) '.html''], ''-helpbrowser''),end'])
      mask Display: plot([-0.05, 1.05, NaN, -0.05, 1.05],[.01, .01, NaN, .99, .99])
  Out1 : Outport
  wires:
  Switch/1 -> Out1/1
  In2/1 -> Switch/3
  In3/1 -> Switch/2
  In1/1 -> Switch/1

== system PCMULib/Standard/Math/Round/mod/mod ==
  In1 : Inport
  In2 : Inport  Port=2
  Mod : Math  Operator=mod  SignedPower=on
  Out1 : Outport
  wires:
  In1/1 -> Mod/1
  Mod/1 -> Out1/1
  In2/1 -> Mod/2

== system PCMULib/Custom/CAN/CanHex2Signed/signal_conditioning/Floor/mod1 ==
  In1 : Inport
  In2 : Inport  Port=2
  Mod : Math  Operator=mod  SignedPower=on
  Out1 : Outport
  wires:
  In1/1 -> Mod/1
  Mod/1 -> Out1/1
  In2/1 -> Mod/2

== system PCMULib/Standard/Discrete dynamics/BumplessRateTransfer/RateLimit/Subsystem1/ESubsystem ==
  Enable_Name : EnablePort
  Constant10 : Constant
      settings: CopyFcn=set_param(gcbh,'ShowName','off');
  Out1 : Outport
  wires:
  Constant10/1 -> Out1/1

== system PCMULib/Standard/Discrete dynamics/BumplessTransfer/LPF1_pole1/Subsystem1/ESubsystem ==
  Enable_Name : EnablePort
  Constant10 : Constant
      settings: CopyFcn=set_param(gcbh,'ShowName','off');
  Out1 : Outport
  wires:
  Constant10/1 -> Out1/1

== stateflow chart PCMULib/Standard/Relation&Logic/Chart ==
